simulink model "Triggered_subsystem_mdl"  (R2021a)
settings: Solver=VariableStepAuto  StartTime=0.0  StopTime=10  FixedStep=0.1  RelTol=1e-3
values from neighbouring files (symbols this model uses):
  ADMM_vec = [ADMM_vec;ADMM_struct]    [Setup.m]
  constraints_struct = [constraints_struct;constraints]    [Setup.m]
  graph = ones(M) - eye(M)    [Setup.m]
  M = size(x0,1)    [Setup.m]
  N = 30    [Setup.m]
  r = [1.0,1.4,0,0,0,0; 0.6,0.4,0,0,0,0; 0,0.9,0,0,0,0; 0,0,1,0,0,0]    [Setup.m]
  T = 0.1    [Setup.m]
  x0 = [0,0.5,0,0,0,0;  0.2,0.9,0,0,0,0; 1.0,0.3,0,0,0,0; 0,0,0,0,0,0]    [Setup.m]
undefined symbols (not defined in the file or in its folder): Acc_from_pos, m, model, MPC_period, N_j, Objective
libraries: dspswit3 x2, uavGuidanceForEachMod x1, simulink x1, dspindex x1
settings Model: Creator=worc4873  LastModifiedBy=lukearcus
settings DebuggingCC: ReadBeforeWriteMsg=DisableAll  WriteAfterWriteMsg=DisableAll  WriteAfterReadMsg=DisableAll  MultiTaskDSMMsg=none
settings ModelReferenceCC: UpdateModelReferenceTargets=IfOutOfDate
settings SFSimCC: SFSimEcho=off

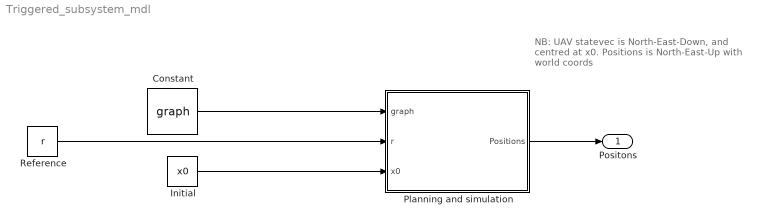
== system Triggered_subsystem_mdl ==
  note: NB: UAV statevec is North-East-Down, and centred at x0. Positions is North-East-Up with world coords
  Constant : Constant  Value=graph
  Initial : Constant  Value=x0
  Planning and simulation : Subsystem
  Reference : Constant  Value=r
  Positons : Outport
  wires:
  Reference/1 -> Planning and simulation/2(r)
  Initial/1 -> Planning and simulation/3(x0)
  Planning and simulation/1(Positions) -> Positons/1
  Constant/1 -> Planning and simulation/1(graph)

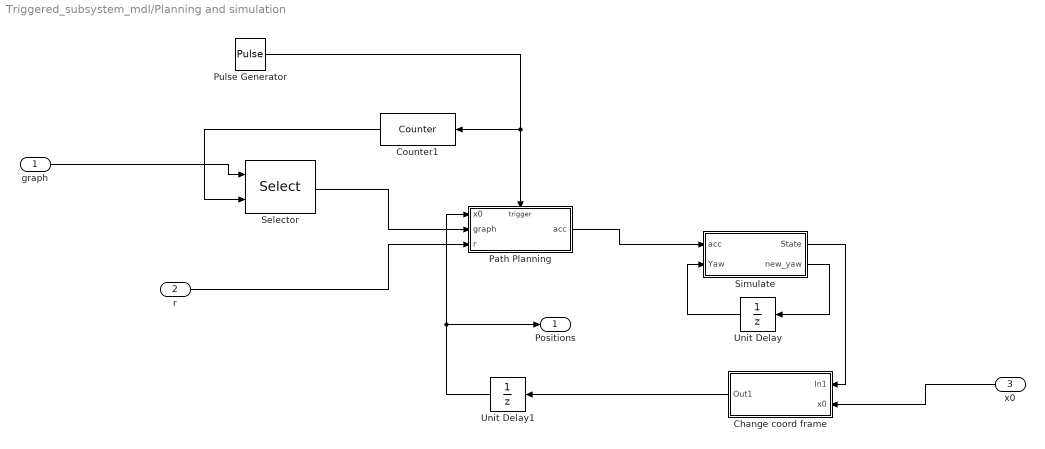
== system Triggered_subsystem_mdl/Planning and simulation ==
  graph : Inport
  r : Inport  Port=2
  x0 : Inport  Port=3
  Change coord frame : Subsystem  TreatAsAtomicUnit=on
  Counter1 : dspswit3/Counter  Direction=Up  CountEvent=Falling edge  CounterSize=User defined  MaxCount=size(graph,3)-1  InitialCount=0  Output=Count  HitValue=32  ResetInput=off  SamplesPerFrame=1  Ts=1  CntDtype=double  HitDtype=Logical
  Path Planning : Subsystem  TreatAsAtomicUnit=on
  Pulse Generator : DiscretePulseGenerator  Period=MPC_period/T  PhaseDelay=1  SampleTime=0.1
  Selector : Selector  NumberOfDimensions=3  IndexMode=Zero-based  InputPortWidth=3  IndexOptions=Select all,Select all,Index vector (port)  Indices=[1 3],1,1  OutputSizes=1,1,1
  Simulate : Subsystem  TreatAsAtomicUnit=on
  Unit Delay : UnitDelay  SampleTime=-1  HasFrameUpgradeWarning=on
  Unit Delay1 : UnitDelay  InitialCondition=x0  SampleTime=-1  HasFrameUpgradeWarning=on
  Positions : Outport
  wires:
  Unit Delay1/1 -> Positions/1, Path Planning/1(x0)
  Simulate/2(new_yaw) -> Unit Delay/1
  Simulate/1(State) -> Change coord frame/1(In1)
  Unit Delay/1 -> Simulate/2(Yaw)
  Pulse Generator/1 -> Counter1/1, Path Planning/Trigger
  Change coord frame/1(Out1) -> Unit Delay1/1
  Path Planning/1(acc) -> Simulate/1(acc)
  r/1 -> Path Planning/3(r)
  x0/1 -> Change coord frame/2(x0)
  graph/1 -> Selector/1
  Selector/1 -> Path Planning/2(graph)
  Counter1/1 -> Selector/2

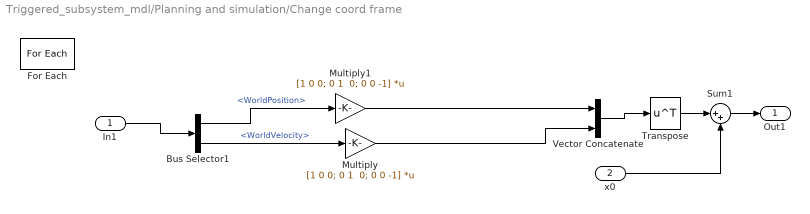
== system Triggered_subsystem_mdl/Planning and simulation/Change coord frame ==
  In1 : Inport  Partition=on  PartitionDimension=2  PartitionWidth=1  PartitionOffset=0
  x0 : Inport  Port=2  Partition=on  PartitionDimension=1  PartitionWidth=1  PartitionOffset=0
  Bus Selector1 : BusSelector  OutputSignals=WorldPosition,WorldVelocity
  For Each : ForEach  DisableCoverage=on
  Multiply : Gain  Gain="[1 0 0; 0 1  0; 0 0 -1]"  Multiplication=Matrix(K*u) (u vector)
  Multiply1 : Gain  Gain="[1 0 0; 0 1  0; 0 0 -1]"  Multiplication=Matrix(K*u) (u vector)
  Sum1 : Sum  Inputs=|++
  Transpose : Math  Operator=transpose  SaturateOnIntegerOverflow=on
  Vector Concatenate : Concatenate
  Out1 : Outport  ConcatenationDimension=1
  wires:
  In1/1 -> Bus Selector1/1
  Bus Selector1/2 -> Multiply/1  "<WorldVelocity>"
  Multiply/1 -> Vector Concatenate/2
  Vector Concatenate/1 -> Transpose/1
  Bus Selector1/1 -> Multiply1/1  "<WorldPosition>"
  Multiply1/1 -> Vector Concatenate/1
  x0/1 -> Sum1/2
  Transpose/1 -> Sum1/1
  Sum1/1 -> Out1/1

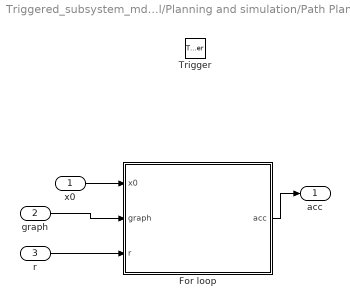
== system Triggered_subsystem_mdl/Planning and simulation/Path Planning ==
  x0 : Inport
  graph : Inport  Port=2
  r : Inport  Port=3
  Trigger : TriggerPort  VariantControl=(inherit)
  For loop : Subsystem  TreatAsAtomicUnit=on
  acc : Outport
  wires:
  x0/1 -> For loop/1(x0)
  graph/1 -> For loop/2(graph)
  r/1 -> For loop/3(r)
  For loop/1(acc) -> acc/1

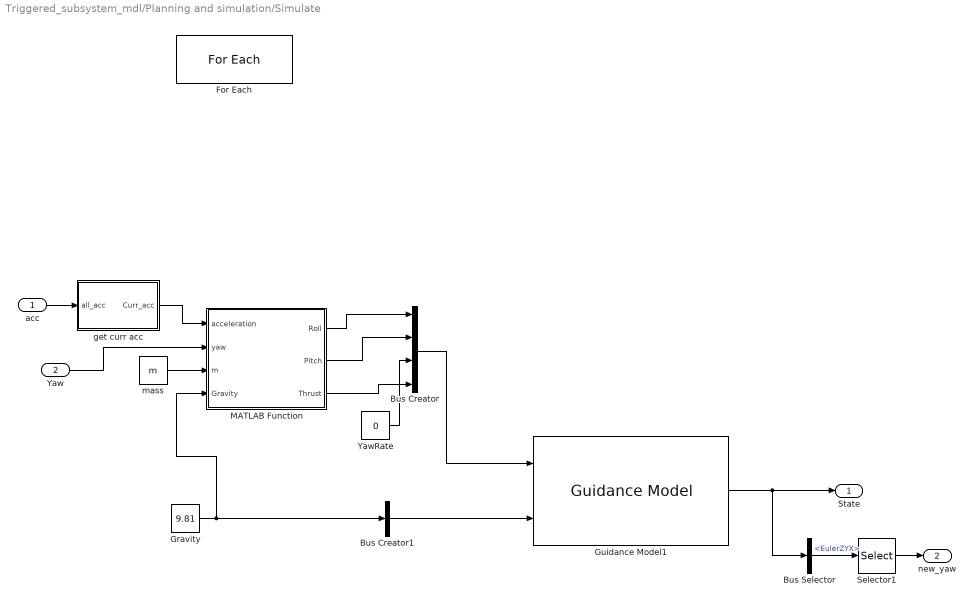
== system Triggered_subsystem_mdl/Planning and simulation/Simulate ==
  acc : Inport  Partition=on  PartitionDimension=2  PartitionWidth=1  PartitionOffset=0
  Yaw : Inport  Port=2  Partition=on  PartitionDimension=2  PartitionWidth=1  PartitionOffset=0
  Bus Creator : BusCreator  Inputs=4  OutDataTypeStr=Bus: MultirotorGuidanceControlBus  NonVirtualBus=on
      settings: InheritFromInputs=off
  Bus Creator1 : BusCreator  Inputs=1  OutDataTypeStr=Bus: MultirotorGuidanceEnvironmentBus  NonVirtualBus=on
      settings: InheritFromInputs=off
  Bus Selector : BusSelector  OutputSignals=EulerZYX
  For Each : ForEach  DisableCoverage=on
  Gravity : Constant  Value=9.81
  Guidance Model1 : uavGuidanceForEachMod/Guidance Model  ModelType=MultirotorGuidance  SpecifiedDataType=double  SimulateUsing=Code generation  InitialWorldPositionMultirotor=[0; 0; 0]  InitialWorldVelocityMultirotor=[0; 0; 0]  InitialEulerZYXMultirotor=[0; 0; 0]  InitialBodyAngularRateRPYMultirotor=[0; 0; 0]  InitialThrustMultirotor=0  InitialNorthFixedWing=0  InitialEastFixedWing=0  InitialHeightFixedWing=0  InitialAirSpeedFixedWing=0  InitialHeadingAngleFixedWing=0  InitialFlightPathAngleFixedWing=0  InitialRollAngleFixedWing=0  InitialRollAngleRateFixedWing=0  PDRollMultirotor=[3402.97,116.67]  PDPitchMultirotor=[3402.97, 116.67]  PYawRateMultirotor=1950  PThrustMultirotor=3900  MassMultirotor=m  PHeightFixedWing=3.9  PHeadingAngleFixedWing=3.9  PFlightPathAngleFixedWing=39  PDRollFixedWing=[3402.97, 116.67]  PAirSpeedFixedWing=1  FlightPathAngleLimitsFixedWing=[-pi/2, pi/2]  StateBusName='MultirotorGuidanceStateBus'  ControlBusName='MultirotorGuidanceControlBus'  EnvironmentBusName='MultirotorGuidanceEnvironmentBus'  DataType=double
  MATLAB Function : MATLAB Function  TreatAsAtomicUnit=on
  Selector1 : Selector  InputPortWidth=3  IndexOptions=Index vector (dialog)  Indices=1  OutputSizes=1
  YawRate : Constant  Value=0
  get curr acc : Subsystem
  mass : Constant  Value=m
  State : Outport  ConcatenationDimension=2
  new_yaw : Outport  Port=2  ConcatenationDimension=2
  wires:
  Guidance Model1/1 -> Bus Selector/1, State/1
  Bus Creator/1 -> Guidance Model1/1
  MATLAB Function/1(Roll) -> Bus Creator/1
  MATLAB Function/2(Pitch) -> Bus Creator/2
  MATLAB Function/3(Thrust) -> Bus Creator/4
  YawRate/1 -> Bus Creator/3
  mass/1 -> MATLAB Function/3(m)
  Yaw/1 -> MATLAB Function/2(yaw)
  Bus Creator1/1 -> Guidance Model1/2
  Gravity/1 -> MATLAB Function/4(Gravity), Bus Creator1/1
  Bus Selector/1 -> Selector1/1  "<EulerZYX>"
  Selector1/1 -> new_yaw/1
  acc/1 -> get curr acc/1(all_acc)
  get curr acc/1(Curr_acc) -> MATLAB Function/1(acceleration)

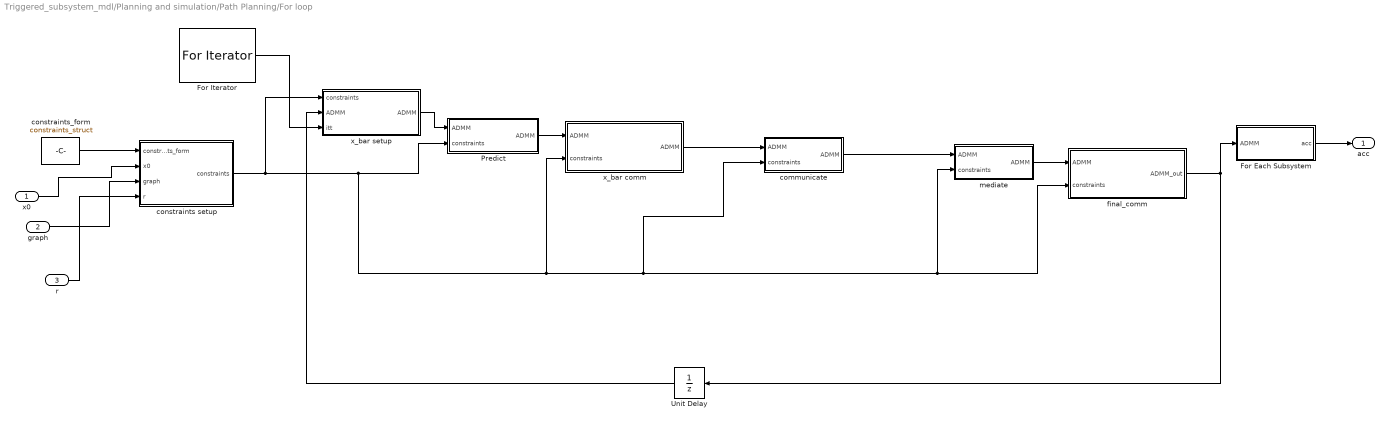
== system Triggered_subsystem_mdl/Planning and simulation/Path Planning/For loop ==
  x0 : Inport
  graph : Inport  Port=2
  r : Inport  Port=3
  For Each Subsystem : Subsystem  TreatAsAtomicUnit=on
  For Iterator : ForIterator  IterationLimit=45
  Predict : Subsystem  TreatAsAtomicUnit=on
  Unit Delay : UnitDelay  InitialCondition=ADMM_vec  SampleTime=-1  HasFrameUpgradeWarning=on
  communicate : Subsystem  TreatAsAtomicUnit=on
  constraints setup : Subsystem  TreatAsAtomicUnit=on
  constraints_form : Constant  Value=constraints_struct  OutDataTypeStr=Bus: constraints
  final_comm : MATLAB Function  TreatAsAtomicUnit=on
  mediate : Subsystem  TreatAsAtomicUnit=on
  x_bar comm : MATLAB Function  TreatAsAtomicUnit=on
  x_bar setup : MATLAB Function  TreatAsAtomicUnit=on
  acc : Outport
  wires:
  constraints_form/1 -> constraints setup/1(constraints_form)
  Predict/1(ADMM) -> x_bar comm/1("ADMM ")
  x_bar comm/1(ADMM) -> communicate/1("ADMM ")
  communicate/1(ADMM) -> mediate/1("ADMM ")
  mediate/1(ADMM) -> final_comm/1(ADMM)
  final_comm/1(ADMM_out) -> Unit Delay/1, For Each Subsystem/1(ADMM)
  For Each Subsystem/1(acc) -> acc/1
  constraints setup/1(constraints) -> x_bar setup/1(constraints), Predict/2(constraints), x_bar comm/2(constraints), final_comm/2(constraints), mediate/2(constraints), communicate/2(constraints)
  x0/1 -> constraints setup/2(x0)
  graph/1 -> constraints setup/3(graph)
  r/1 -> constraints setup/4(r)
  For Iterator/1 -> x_bar setup/3(itt)
  Unit Delay/1 -> x_bar setup/2("ADMM ")
  x_bar setup/1(ADMM) -> Predict/1("ADMM ")

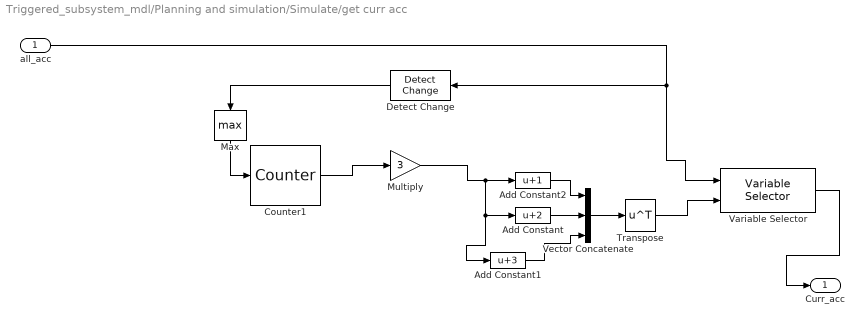
== system Triggered_subsystem_mdl/Planning and simulation/Simulate/get curr acc ==
  all_acc : Inport
  Add Constant : Bias  Bias=2
  Add Constant1 : Bias  Bias=3
  Add Constant2 : Bias  Bias=1
  Counter1 : dspswit3/Counter  Direction=Up  CountEvent=Free running  CounterSize=User defined  MaxCount=30  InitialCount=0  Output=Count  HitValue=32  ResetInput=on  SamplesPerFrame=1  Ts=0.1  CntDtype=double  HitDtype=Logical
  Detect Change : simulink/Logic and Bit Operations/Detect Change  vinit=0  OutDataTypeStr=boolean
  Max : MinMax  Function=max
  Multiply : Gain  Gain=3
  Transpose : Math  Operator=transpose  SaturateOnIntegerOverflow=on
  Variable Selector : dspindex/Variable Selector  NumInputs=1  rowsOrCols=Rows  IdxMode=Variable  Elements=[1 3]  ZerOneIdxMode=One-based  errmode=Clip Index  FillMode=on  FillValues=0
  Vector Concatenate : Concatenate  NumInputs=3
  Curr_acc : Outport
  wires:
  Detect Change/1 -> Max/1
  Transpose/1 -> Variable Selector/2
  Vector Concatenate/1 -> Transpose/1
  Multiply/1 -> Add Constant1/1, Add Constant/1, Add Constant2/1
  Variable Selector/1 -> Curr_acc/1
  all_acc/1 -> Variable Selector/1, Detect Change/1
  Counter1/1 -> Multiply/1
  Add Constant2/1 -> Vector Concatenate/1
  Max/1 -> Counter1/1
  Add Constant1/1 -> Vector Concatenate/3
  Add Constant/1 -> Vector Concatenate/2

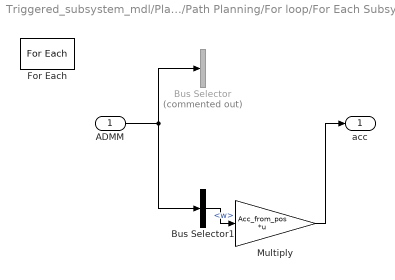
== system Triggered_subsystem_mdl/Planning and simulation/Path Planning/For loop/For Each Subsystem ==
  ADMM : Inport  Partition=on  PartitionDimension=1  PartitionWidth=1  PartitionOffset=0
  Bus Selector : BusSelector  Commented=on  OutputSignals=u
  Bus Selector1 : BusSelector  OutputSignals=w
  For Each : ForEach  DisableCoverage=on
  Multiply : Gain  Gain=Acc_from_pos  Multiplication=Matrix(K*u) (u vector)
  acc : Outport  ConcatenationDimension=2
  wires:
  ADMM/1 -> Bus Selector/1, Bus Selector1/1
  Bus Selector1/1 -> Multiply/1  "<w>"
  Multiply/1 -> acc/1

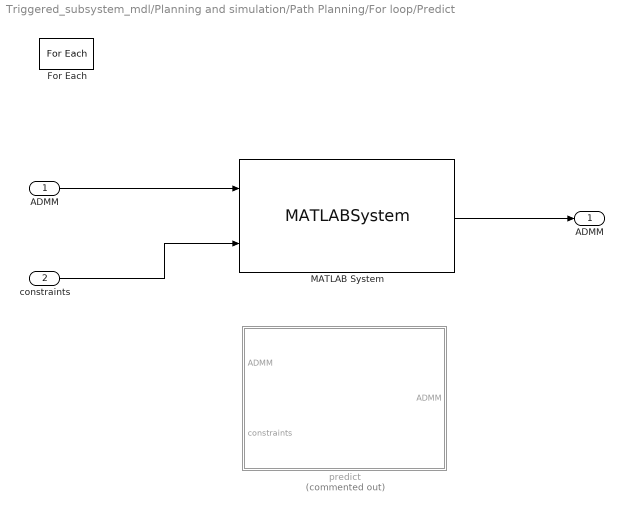
== system Triggered_subsystem_mdl/Planning and simulation/Path Planning/For loop/Predict ==
  "ADMM " : Inport  OutDataTypeStr=Bus: ADMM  Partition=on  PartitionDimension=1  PartitionWidth=1  PartitionOffset=0
  constraints : Inport  Port=2  OutDataTypeStr=Bus: constraints  Partition=on  PartitionDimension=1  PartitionWidth=1  PartitionOffset=0
  For Each : ForEach  DisableCoverage=on
  MATLAB System : MATLABSystem  System=predictADMM  N=N  delta=delta  M=M  SampleTime=T  OffsetTime=0.05  TickTime=0.1  SimulateUsing=Interpreted execution
      mask Type: predictADMM
      mask Display:
      | disp('predictADMM');
      | port_label('input',1,'ADMM_input');
      | port_label('input',2,'constraints');
      | port_label('output',1,'ADMM_update');
  predict : MATLAB Function  Commented=on  TreatAsAtomicUnit=on
  ADMM : Outport  ConcatenationDimension=1
  wires:
  constraints/1 -> MATLAB System/2
  "ADMM "/1 -> MATLAB System/1
  MATLAB System/1 -> ADMM/1

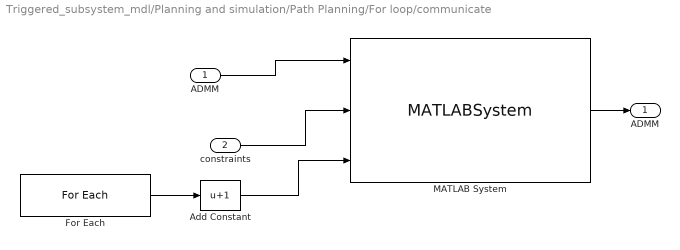
== system Triggered_subsystem_mdl/Planning and simulation/Path Planning/For loop/communicate ==
  "ADMM " : Inport  OutDataTypeStr=Bus: ADMM  Partition=on  PartitionDimension=1  PartitionWidth=1  PartitionOffset=0
  constraints : Inport  Port=2  OutDataTypeStr=Bus: constraints  Partition=on  PartitionDimension=1  PartitionWidth=1  PartitionOffset=0
  Add Constant : Bias  Bias=1
  For Each : ForEach  DisableCoverage=on  ShowIterationIndex=on
  MATLAB System : MATLABSystem  System=CoordinateADMM  N=N  delta=delta  M=M  SampleTime=T  OffsetTime=0.05  TickTime=0.1  SimulateUsing=Interpreted execution
      mask Type: CoordinateADMM
      mask Display:
      | disp('CoordinateADMM');
      | port_label('input',1,'ADMM_input');
      | port_label('input',2,'constraints');
      | port_label('input',3,'i');
      | port_label('output',1,'ADMM_update');
  ADMM : Outport  ConcatenationDimension=1
  wires:
  "ADMM "/1 -> MATLAB System/1
  constraints/1 -> MATLAB System/2
  MATLAB System/1 -> ADMM/1
  For Each/1 -> Add Constant/1
  Add Constant/1 -> MATLAB System/3

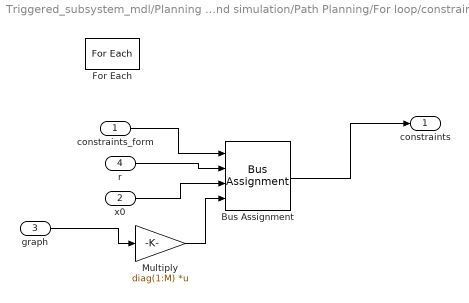
== system Triggered_subsystem_mdl/Planning and simulation/Path Planning/For loop/constraints setup ==
  constraints_form : Inport  Partition=on  PartitionDimension=1  PartitionWidth=1  PartitionOffset=0
  x0 : Inport  Port=2  Partition=on  PartitionDimension=1  PartitionWidth=1  PartitionOffset=0
  graph : Inport  Port=3  Partition=on  PartitionDimension=1  PartitionWidth=1  PartitionOffset=0
  r : Inport  Port=4  Partition=on  PartitionDimension=1  PartitionWidth=1  PartitionOffset=0
  Bus Assignment : BusAssignment  AssignedSignals=r,x0,N_j
  For Each : ForEach  DisableCoverage=on
  Multiply : Gain  Gain=diag(1:M)  Multiplication=Matrix(K*u) (u vector)
  constraints : Outport  ConcatenationDimension=1
  wires:
  constraints_form/1 -> Bus Assignment/1
  Bus Assignment/1 -> constraints/1
  r/1 -> Bus Assignment/2
  x0/1 -> Bus Assignment/3
  graph/1 -> Multiply/1
  Multiply/1 -> Bus Assignment/4

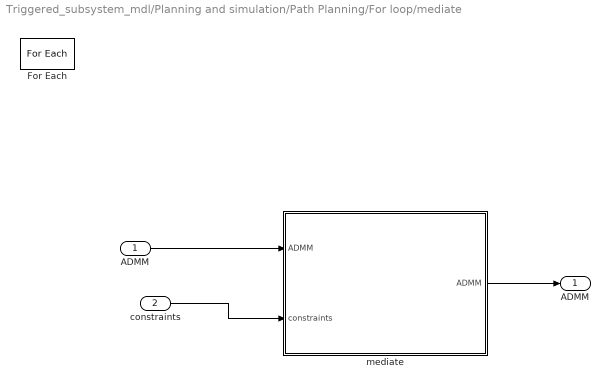
== system Triggered_subsystem_mdl/Planning and simulation/Path Planning/For loop/mediate ==
  "ADMM " : Inport  Partition=on  PartitionDimension=1  PartitionWidth=1  PartitionOffset=0
  constraints : Inport  Port=2  Partition=on  PartitionDimension=1  PartitionWidth=1  PartitionOffset=0
  For Each : ForEach  DisableCoverage=on
  mediate : MATLAB Function  TreatAsAtomicUnit=on
  ADMM : Outport  ConcatenationDimension=1
  wires:
  "ADMM "/1 -> mediate/1("ADMM ")
  constraints/1 -> mediate/2(constraints)
  mediate/1(ADMM) -> ADMM/1

== matlab function Triggered_subsystem_mdl/Planning and simulation/Path Planning/For loop/Predict/predict ==
  data: ADMM input Bus: ADMM; ADMM output; Objective parameter; model parameter; constraints input Bus: constraints
function ADMM = predict_step(ADMM,Objective, model, constraints)

Q = Objective.Q;
R = Objective.R;
N = Objective.N;

Nd = 3;
nx = size(Q,1);
nu = size(R,1);

A = model.A;
B = model.B;
umax = model.umax;
umin = model.umin;


N_j = constraints.N_j;
r = constraints.r;
x0 = constraints.x0;

rho = ADMM.rho;
lambda = ADMM.lambda;
lambda_from_j = ADMM.lambda_from_j;
w = ADMM.w;
w_from_j = ADMM.w_from_j;

min_input = repmat(ones(nu,1)*umin,N,1);
max_input = repmat(ones(nu,1)*umax,N,1);
% - linear dynamics

u_bound = [inf((N+1)*nx,1);max_input];
l_bound = [-inf((N+1)*nx,1);min_input];


posM = blkdiag(eye(Nd),zeros(nx-Nd)); % Matrix to take only position from the state vector x (zeros rest)
d = [eye(Nd),zeros(Nd,nx-Nd)]; % Matrix to take only position from the state vector x (only returns pos)
posMN = kron(eye(N+1),d); %returns pos across time steps

Ax = kron(speye(N+1), -speye(nx)) + kron(sparse(diag(ones(N, 1), -1)), A);
Bu = kron([sparse(1, N); speye(N)], B);
Aeq = [Ax, Bu];
b_eq = [-x0'; zeros(N*nx, 1)];
P_new = blkdiag( kron(eye(N), Q+ (size(N_j,2)+1)*rho/2*posM ), Q+(size(N_j,2)+1)*rho/2*posM, kron(eye(N), R) );

q = prediction_linear(lambda,lambda_from_j,w,w_from_j,rho,r',Q,N,nu,posMN);

qp_opts = optimoptions('quadprog','Display','off','Algorithm','active-set');
init = [ADMM.x;ADMM.u];
res = quadprog(P_new,q,[],[], full(Aeq),b_eq,l_bound,u_bound,init,qp_opts);
ADMM.x = res(1:nx*(N+1));
ADMM.u = res((N+1)*nx+1:end);

end

== matlab function Triggered_subsystem_mdl/Planning and simulation/Path Planning/For loop/x_bar comm ==
  data: ADMM input Bus: ADMM; ADMM output; constraints input Bus: constraints
function ADMM = comm_xbar(ADMM,constraints)

for i =1:size(ADMM,1)
    ADMM(i).x_bar(:,i) = ADMM(i).x;
    nonzero_N_j = nonzeros(constraints(i).N_j);
    for j = 1:nnz(constraints(i).N_j)
        ADMM(i).x_bar(:,nonzero_N_j(j)) = ADMM(nonzero_N_j(j)).x;
    end
end

end

== matlab function Triggered_subsystem_mdl/Planning and simulation/Path Planning/For loop/final_comm ==
  data: ADMM input Bus: ADMM; ADMM_out output Bus: ADMM; constraints input Bus: constraints
function ADMM_out = final_comm(ADMM,constraints)
    
ADMM_out = ADMM;
    for i = 1:size(ADMM_out,1)
        nonzero_N_j = nonzeros(constraints(i).N_j);
        for j = 1:nnz(constraints(i).N_j)
            curr_comm = nonzero_N_j(j);
            ADMM_out(i).lambda_from_j(:,nonzero_N_j(j)) = ADMM_out(curr_comm).lambda_to_j(:,i);
            ADMM_out(i).w_from_j(:,nonzero_N_j(j)) = ADMM_out(curr_comm).w_to_j(:,i);
        end
        
    end
    
end

== matlab function Triggered_subsystem_mdl/Planning and simulation/Path Planning/For loop/mediate/mediate ==
  data: ADMM input Bus: ADMM; ADMM output; N parameter; constraints input Bus: constraints
function ADMM = mediate_step(ADMM,N, constraints)

Nd = 3;
nx = size(ADMM.x,1)/(N+1);

d = [eye(Nd),zeros(Nd,nx-Nd)]; % Matrix to take only position from the state vector x (only returns pos)
posMN = kron(eye(N+1),d); %returns pos across time steps


ADMM.lambda = ADMM.lambda + ADMM.rho * (posMN * ADMM.x-ADMM.w);
nonzero_N_j = nonzeros(constraints.N_j);
for j = 1:nnz(constraints.N_j)
    ADMM.lambda_to_j(:,nonzero_N_j(j)) = ADMM.lambda_to_j(:,nonzero_N_j(j)) + ADMM.rho * (posMN*ADMM.x_bar(:,nonzero_N_j(j)) - ADMM.w_to_j(:,nonzero_N_j(j)));
end

end

== matlab function Triggered_subsystem_mdl/Planning and simulation/Simulate/MATLAB Function ==
  data: Roll output; Pitch output; acceleration input; Thrust output; yaw input; m input; Gravity input
function [Roll,Pitch,Thrust] = acc_to_input(acceleration,yaw,m,Gravity)

 
    Pitch = atan2((-acceleration(1)*cos(yaw)-acceleration(2)*sin(yaw)), (acceleration(3) + Gravity));
    Roll = atan2(((-acceleration(1)*sin(yaw)+acceleration(2)*cos(yaw))*cos(Pitch)), (acceleration(3)+Gravity));
    
    Thrust = m*(acceleration(3)+Gravity)/(cos(Pitch)*cos(Roll));

end

== matlab function Triggered_subsystem_mdl/Planning and simulation/Path Planning/For loop/x_bar setup ==
  data: constraints input Bus: constraints; ADMM output; ADMM input Bus: ADMM; Objective parameter; model parameter; itt input
function ADMM = fcn(constraints,ADMM,Objective, model, itt)

if itt == 1
    nx = size(Objective.Q,2);
    nu = size(Objective.R,1);
    N = Objective.N;
    M = size(ADMM,1);
    
    x_init = zeros(nx*(N+1),M);
    u_init = zeros(nu*N,M);
    for i = 1:M
%         Ax = kron(speye(N+1), -speye(nx)) + kron(sparse(diag(ones(N, 1), -1)), model.A);
%         Bu = kron([sparse(1, N); speye(N)], model.B);
%         b_eq = [-constraints(i).x0 zeros(1, N*nx)]';
        [x_init(:,i),u_init(:,i)] = init_traj(ADMM(i).rho,Objective,constraints(i),model); %initial solution
%         init_vel = constraints(i).x0(4:6)';
%         T = model.B(4,1);
%         steps = round(max(abs(init_vel))/(T*model.umax));
%         steps = min(steps,N);
%         if steps >= 1
%             u_start = model.umax/max(abs(init_vel))*-init_vel;
%             final_vel = init_vel + T*(steps-1)*u_start;
%             u_start = repmat(u_start,steps-1,1);
%             u_start = [u_start;-final_vel/T];
%         else
%             u_start = [];
%         end
%         u_init(:,i) = [u_start;zeros(N*nu-size(u_start,1),1)];
%         x_init(:,i) = (Ax)\(b_eq - Bu*u_init(:,i));
%         direction = constraints(i).r(1:3)'-x_init(nx*N+1:nx*N+3,i);
%         start = floor((N-size(u_start,1)/nu)/2);
%         for k = 1:100
%             
%             accel = (model.umax/max(abs(direction)))*direction;
%             u_init(steps*nu+1:(steps+start)*nu,i) = repmat(accel,start,1);
%             if steps+2*start < N
%                 u_init((steps+start)*nu+1:(steps+2*start)*nu,i) = -repmat(accel,start,1);
%             else
%                 u_init((steps+start)*nu+1:end,i) = -repmat(accel, N-steps-start,1);
%             end
%             x_init(:,i) = (Ax)\(b_eq - Bu*u_init(:,i));
%             
%             final_diff = constraints(i).r(1:3)'-x_init(nx*N+1:nx*N+3,i);
%             final_diff = final_diff';
%             
%             if norm(x_init(nx*N+1:end,i)-constraints(i).r') < 0.1
%                 break;
%             elseif sign(dot(final_diff,direction)) ~= 1
%                 start = start - 1;
%                 u_init(:,i) = [u_start;zeros(N*nu-size(u_start,1),1)];
%                 x_init(:,i) = (Ax)\(b_eq - Bu*u_init(:,i));
%             else
%                 break;
%             end
%         end
        %accel in direction of target, then max deccel, start deccel at N/2
        %and tune from there
    end
    for i =1:M
        ADMM(i).x = x_init(:,i);
        ADMM(i).u = u_init(:,i);
        ADMM(i).x_bar(:,i) = x_init(:,i);
        nonzero_N_j = nonzeros(constraints(i).N_j);
        for j = 1:nnz(constraints(i).N_j)
            ADMM(i).x_bar(:,nonzero_N_j(j)) = x_init(:,nonzero_N_j(j));
        end
    end
end

end
